simulink model "intersample_ripple"  (R2021b)
settings: Solver=VariableStepAuto  StartTime=0.0  StopTime=10.0  RelTol=1e-3
undefined symbols (not defined in the file): Ts
libraries: cstblocks x2
settings Model: Creator=varunsampat  LastModifiedBy=varunsampat

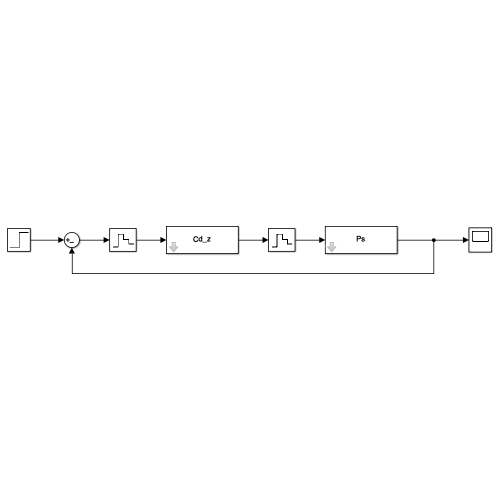
[thumbnail: Simulink's stored preview of the top-level diagram]
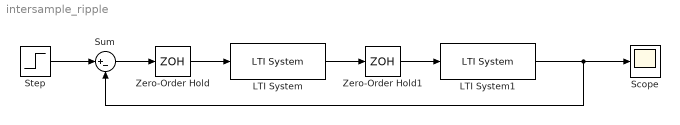
== system intersample_ripple ==
  LTI System : cstblocks/LTI System  sys=Cd_z  IC=[]
  LTI System1 : cstblocks/LTI System  sys=Ps  IC=[]
  Scope : Scope
  Step : Step  SampleTime=0
  Sum : Sum  Inputs=|+-
  Zero-Order Hold : ZeroOrderHold  SampleTime=Ts
  Zero-Order Hold1 : ZeroOrderHold  SampleTime=Ts
  wires:
  Zero-Order Hold/1 -> LTI System/1
  LTI System/1 -> Zero-Order Hold1/1
  Zero-Order Hold1/1 -> LTI System1/1
  LTI System1/1 -> Sum/2, Scope/1
  Step/1 -> Sum/1
  Sum/1 -> Zero-Order Hold/1
